simulink model "Hysteresis"  (R2021b)
settings: Solver=VariableStepAuto  StartTime=0.0  StopTime=10.0  RelTol=1e-3
settings Model: Creator=t  LastModifiedBy=t

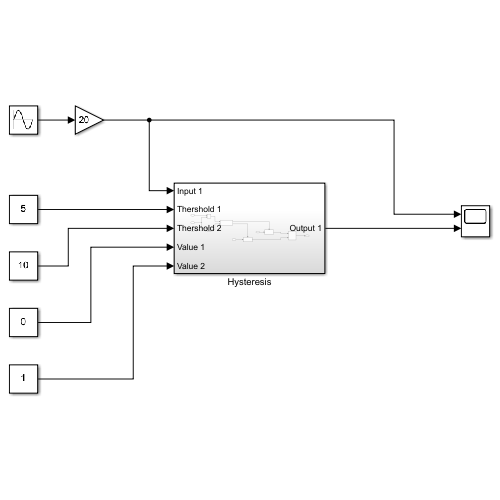
[thumbnail: Simulink's stored preview of the top-level diagram]
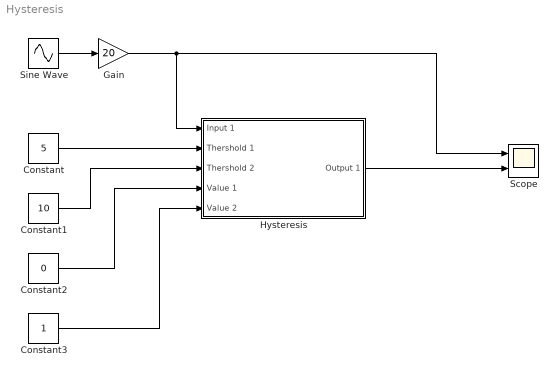
== system Hysteresis ==
  Constant : Constant  Value=5
  Constant1 : Constant  Value=10
  Constant2 : Constant  Value=0
  Constant3 : Constant
  Gain : Gain  Gain=20
  Hysteresis : Subsystem
  Scope : Scope  NumInputPorts=2
  Sine Wave : Sin  SampleTime=0
  wires:
  Constant/1 -> Hysteresis/2(Thershold 1)
  Constant1/1 -> Hysteresis/3(Thershold 2)
  Constant2/1 -> Hysteresis/4(Value 1)
  Constant3/1 -> Hysteresis/5(Value 2)
  Sine Wave/1 -> Gain/1
  Gain/1 -> Scope/1, Hysteresis/1(Input 1)
  Hysteresis/1(Output 1) -> Scope/2

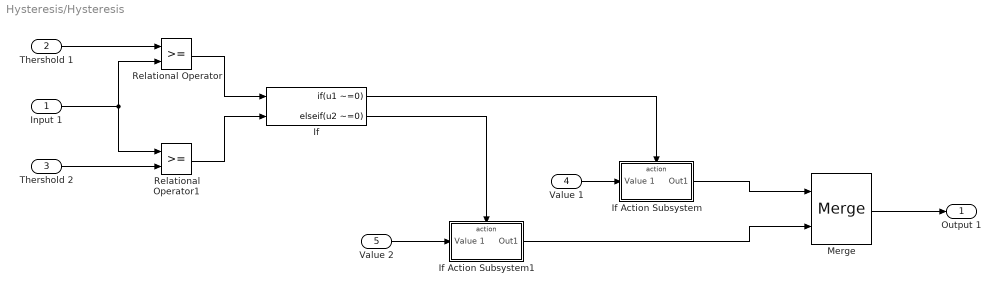
== system Hysteresis/Hysteresis ==
  Input 1 : Inport
  Thershold 1 : Inport  Port=2
  Thershold 2 : Inport  Port=3
  Value 1 : Inport  Port=4
  Value 2 : Inport  Port=5
  If : If  NumInputs=2  IfExpression=u1 ~=0  ElseIfExpressions=u2 ~=0  ShowElse=off
  If Action Subsystem : Subsystem  TreatAsAtomicUnit=on
  If Action Subsystem1 : Subsystem  TreatAsAtomicUnit=on
  Merge : Merge
  Relational Operator : RelationalOperator  OutDataTypeStr=boolean  RndMeth=Simplest
  Relational Operator1 : RelationalOperator  OutDataTypeStr=boolean  RndMeth=Simplest
  Output 1 : Outport
  wires:
  Input 1/1 -> Relational Operator1/1, Relational Operator/2
  Value 1/1 -> If Action Subsystem/1(Value 1)
  If/1 -> If Action Subsystem/Action
  Relational Operator1/1 -> If/2
  Value 2/1 -> If Action Subsystem1/1(Value 1)
  If Action Subsystem1/1(Out1) -> Merge/2
  Thershold 2/1 -> Relational Operator1/2
  If/2 -> If Action Subsystem1/Action
  Merge/1 -> Output 1/1
  If Action Subsystem/1(Out1) -> Merge/1
  Relational Operator/1 -> If/1
  Thershold 1/1 -> Relational Operator/1

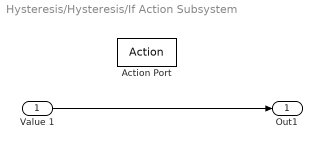
== system Hysteresis/Hysteresis/If Action Subsystem ==
  Value 1 : Inport
  Action Port : ActionPort  ActionPortLabel=if(u1 ~=0)
  Out1 : Outport
  wires:
  Value 1/1 -> Out1/1

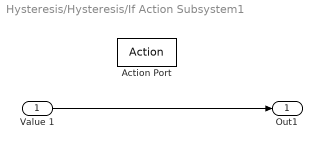
== system Hysteresis/Hysteresis/If Action Subsystem1 ==
  Value 1 : Inport
  Action Port : ActionPort  ActionPortLabel=elseif(u2 ~=0)
  Out1 : Outport
  wires:
  Value 1/1 -> Out1/1
